simulink model "CartNPendulum"  (R2025a)
settings: Solver=VariableStepAuto  StartTime=0.0  StopTime=10.0  RelTol=1e-3
libraries: rllib x3
settings Model: Creator=tanayraghunandansrinivasa  LastModifiedBy=tanayraghunandansrinivasa

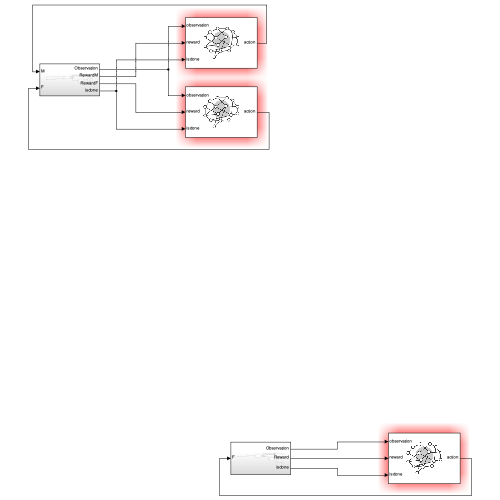
[thumbnail: Simulink's stored preview of the top-level diagram]
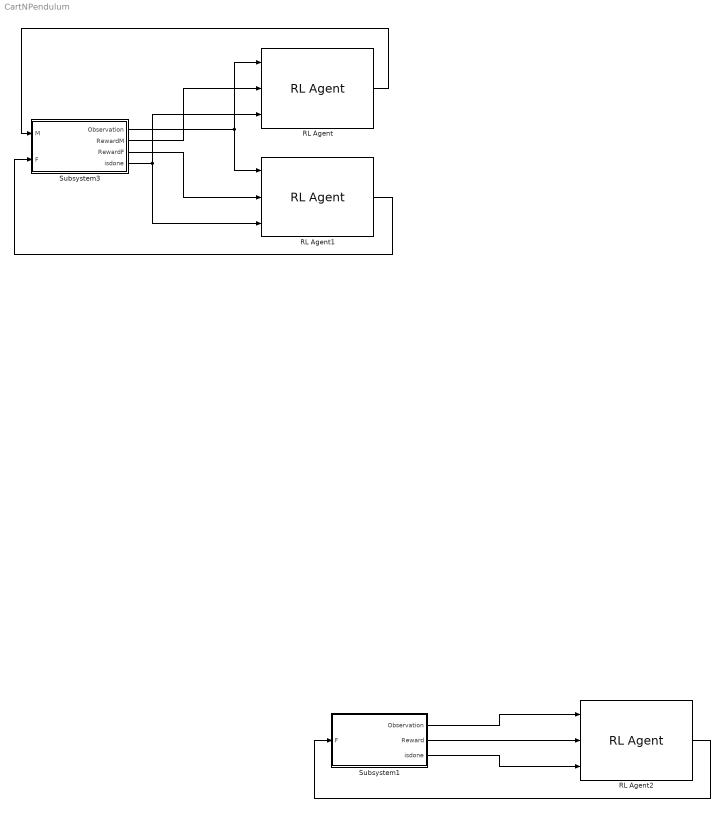
== system CartNPendulum ==
  RL Agent : rllib/RL Agent  Agent=agentObj  ExternalActionAsInput=off  ProvideLastAction=off  ProvideCumRwd=off  TreatAsDirectFeedthrough=on  UseStrictObservationDataTypes=off
  RL Agent1 : rllib/RL Agent  Agent=agentObj  ExternalActionAsInput=off  ProvideLastAction=off  ProvideCumRwd=off  TreatAsDirectFeedthrough=on  UseStrictObservationDataTypes=off
  RL Agent2 : rllib/RL Agent  Agent=agentObj  ExternalActionAsInput=off  ProvideLastAction=off  ProvideCumRwd=off  TreatAsDirectFeedthrough=on  UseStrictObservationDataTypes=off
  Subsystem1 : Subsystem
  Subsystem3 : Subsystem
  wires:
  Subsystem3/1(Observation) -> RL Agent1/1, RL Agent/1
  Subsystem3/2(RewardM) -> RL Agent/2
  Subsystem3/4(isdone) -> RL Agent/3, RL Agent1/3
  RL Agent/1 -> Subsystem3/1(M)
  Subsystem3/3(RewardF) -> RL Agent1/2
  RL Agent1/1 -> Subsystem3/2(F)
  Subsystem1/1(Observation) -> RL Agent2/1
  Subsystem1/3(isdone) -> RL Agent2/3
  Subsystem1/2(Reward) -> RL Agent2/2
  RL Agent2/1 -> Subsystem1/1(F)

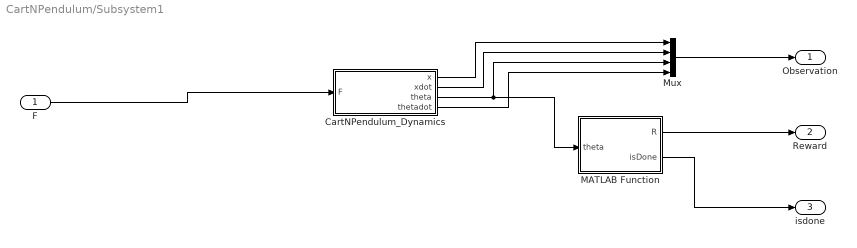
== system CartNPendulum/Subsystem1 ==
  F : Inport
  CartNPendulum_Dynamics : Subsystem
  MATLAB Function : MATLAB Function  TreatAsAtomicUnit=on
  Mux : Mux
  Observation : Outport
  Reward : Outport  Port=2
  isdone : Outport  Port=3
  wires:
  F/1 -> CartNPendulum_Dynamics/1(F)
  CartNPendulum_Dynamics/1(x) -> Mux/1
  CartNPendulum_Dynamics/2(xdot) -> Mux/2
  CartNPendulum_Dynamics/3(theta) -> Mux/3, MATLAB Function/1(theta)
  CartNPendulum_Dynamics/4(thetadot) -> Mux/4
  Mux/1 -> Observation/1
  MATLAB Function/1(R) -> Reward/1
  MATLAB Function/2(isDone) -> isdone/1

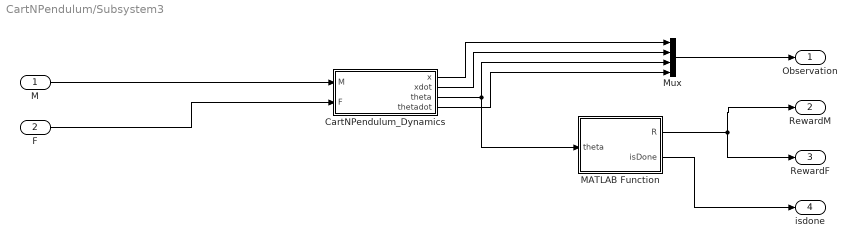
== system CartNPendulum/Subsystem3 ==
  M : Inport
  F : Inport  Port=2
  CartNPendulum_Dynamics : Subsystem
  MATLAB Function : MATLAB Function  TreatAsAtomicUnit=on
  Mux : Mux
  Observation : Outport
  RewardM : Outport  Port=2
  RewardF : Outport  Port=3
  isdone : Outport  Port=4
  wires:
  M/1 -> CartNPendulum_Dynamics/1(M)
  F/1 -> CartNPendulum_Dynamics/2(F)
  CartNPendulum_Dynamics/1(x) -> Mux/1
  CartNPendulum_Dynamics/2(xdot) -> Mux/2
  CartNPendulum_Dynamics/3(theta) -> Mux/3, MATLAB Function/1(theta)
  CartNPendulum_Dynamics/4(thetadot) -> Mux/4
  Mux/1 -> Observation/1
  MATLAB Function/1(R) -> RewardM/1, RewardF/1
  MATLAB Function/2(isDone) -> isdone/1

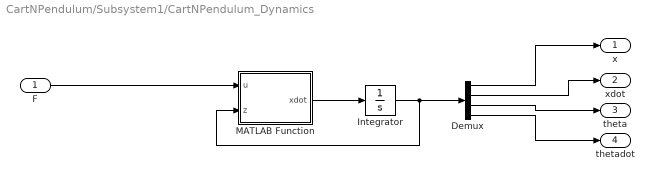
== system CartNPendulum/Subsystem1/CartNPendulum_Dynamics ==
  F : Inport
  Demux : Demux
  Integrator : Integrator
  MATLAB Function : MATLAB Function  TreatAsAtomicUnit=on
  x : Outport
  xdot : Outport  Port=2
  theta : Outport  Port=3
  thetadot : Outport  Port=4
  wires:
  F/1 -> MATLAB Function/1(u)
  MATLAB Function/1(xdot) -> Integrator/1
  Integrator/1 -> MATLAB Function/2(z), Demux/1
  Demux/1 -> x/1
  Demux/2 -> xdot/1
  Demux/3 -> theta/1
  Demux/4 -> thetadot/1

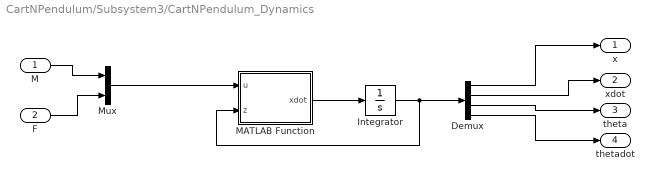
== system CartNPendulum/Subsystem3/CartNPendulum_Dynamics ==
  M : Inport
  F : Inport  Port=2
  Demux : Demux
  Integrator : Integrator
  MATLAB Function : MATLAB Function  TreatAsAtomicUnit=on
  Mux : Mux  Inputs=2
  x : Outport
  xdot : Outport  Port=2
  theta : Outport  Port=3
  thetadot : Outport  Port=4
  wires:
  M/1 -> Mux/1
  F/1 -> Mux/2
  Mux/1 -> MATLAB Function/1(u)
  MATLAB Function/1(xdot) -> Integrator/1
  Integrator/1 -> MATLAB Function/2(z), Demux/1
  Demux/1 -> x/1
  Demux/2 -> xdot/1
  Demux/3 -> theta/1
  Demux/4 -> thetadot/1

== matlab function CartNPendulum/Subsystem3/MATLAB Function ==
  data: theta input; R output; isDone output
function [R, isDone] = fcn(theta)
    if theta > 30
        R = -10;
        isDone = true;
    else
        R = 10/0.01;
        isDone = false;
    end
end

== matlab function CartNPendulum/Subsystem3/CartNPendulum_Dynamics/MATLAB Function ==
  data: u input; xdot output; z input
function xdot = fcn(u ,z)

    % State variables: [x, xdot, theta, thetadot]
    x = z(1);
    xdot = z(2);
    theta = z(3);
    thetadot = z(4);

    % Unpacking Parameters
    mp = p.mp; mc = p.mc; d = p.d; g = p.g; I = p.I; 
    rated_torque = p.rated_torque; b = p.b; 
    rated_torque_cart = p.rated_torque_cart;

    M = u(1);
    F = u(2);
    
    % Clip Control Inputs
    M = max(min(M, rated_torque), -rated_torque);
    F = max(min(F, rated_torque_cart), -rated_torque_cart);

    % Defining Equations of Motion
    xddot = (I*F + d^2*mp*F - I*b*xdot - b*d^2*mp*xdot - d^3*mp^2*thetadot^2*sin(theta) ...
             + d*mp*M*cos(theta) + d^2*g*mp^2*cos(theta)*sin(theta) - I*d*mp*thetadot^2*sin(theta)) ...
            / (I*mc + I*mp + d^2*mp^2 - d^2*mp^2*cos(theta)^2 + d^2*mc*mp);

    thetaddot = (mc*M + mp*M + d*mp*F*cos(theta) + d*g*mp^2*sin(theta) - d^2*mp^2*thetadot^2*cos(theta)*sin(theta) ...
                 - b*d*mp*xdot*cos(theta) + d*g*mc*mp*sin(theta)) ...
                / (I*mc + I*mp + d^2*mp^2 - d^2*mp^2*cos(theta)^2 + d^2*mc*mp);

    % State Derivatives
    zdot(1) = z(2);
    zdot(2) = xddot;
    zdot(3) = z(4);
    zdot(4) = thetaddot;
    
    zdot = zdot';
end

== matlab function CartNPendulum/Subsystem1/CartNPendulum_Dynamics/MATLAB Function ==
  data: u input; xdot output; z input
function xdot = fcn(u ,z)

    % State variables: [x, xdot, theta, thetadot]
    x = z(1);
    xdot = z(2);
    theta = z(3);
    thetadot = z(4);

    % Unpacking Parameters
    mp = p.mp; mc = p.mc; d = p.d; g = p.g; I = p.I; 
    rated_torque = p.rated_torque; b = p.b; 
    rated_torque_cart = p.rated_torque_cart;

    F = u;
    M = 0;
    
    % Clip Control Inputs
    M = max(min(M, rated_torque), -rated_torque);
    F = max(min(F, rated_torque_cart), -rated_torque_cart);

    % Defining Equations of Motion
    xddot = (I*F + d^2*mp*F - I*b*xdot - b*d^2*mp*xdot - d^3*mp^2*thetadot^2*sin(theta) ...
             + d*mp*M*cos(theta) + d^2*g*mp^2*cos(theta)*sin(theta) - I*d*mp*thetadot^2*sin(theta)) ...
            / (I*mc + I*mp + d^2*mp^2 - d^2*mp^2*cos(theta)^2 + d^2*mc*mp);

    thetaddot = (mc*M + mp*M + d*mp*F*cos(theta) + d*g*mp^2*sin(theta) - d^2*mp^2*thetadot^2*cos(theta)*sin(theta) ...
                 - b*d*mp*xdot*cos(theta) + d*g*mc*mp*sin(theta)) ...
                / (I*mc + I*mp + d^2*mp^2 - d^2*mp^2*cos(theta)^2 + d^2*mc*mp);

    % State Derivatives
    zdot(1) = z(2);
    zdot(2) = xddot;
    zdot(3) = z(4);
    zdot(4) = thetaddot;
    
    zdot = zdot';
end

== matlab function CartNPendulum/Subsystem1/MATLAB Function ==
  data: theta input; R output; isDone output
function [R, isDone] = fcn(theta)
    if theta > 30
        R = -10;
        isDone = true;
    else
        R = 10/0.01;
        isDone = false;
    end
end
